simulink model "WinchDynamicsAndControl"  (R2020a)
settings: Solver=FixedStepAuto  StartTime=0.0  StopTime=simInit.TSIM  MaxStep=0.01  RelTol=1e-1
InitFcn:
  | close all
undefined symbols (not defined in the file): constr, DiscIntNeverNeededParam, params, simInit, winchParameter
libraries: simulink x4
Description:
  | % Copyright 2020 Delft University of Technology
  | %
  | % Licensed under the Apache License, Version 2.0 (the "License");
  | % you may not use this file except in compliance with the License.
  | % You may obtain a copy of the License at
  | %
  | %      http://www.apache.org/licenses/LICENSE-2.0
  | %
  | % Unless required by applicable law or agreed to in writing, software
  | % distributed under the License is distributed on an "AS IS" BASIS,
  | % WITHOUT WARRANTIES OR CONDITIONS OF ANY KIND, either express or implied.
  | % See the License for the specific language governing permissions and
  | % limitations under the License.
settings Model: ExtModeTrigDuration=100  Creator=Sebastian  LastModifiedBy=dylaneijkelhof
settings SolverCC: SolverJacobianMethodControl=FullAnalytical
settings DataIOCC: SaveFormat=Array  SaveOutput=off  DSMLogging=off  SaveTime=off  ReturnWorkspaceOutputs=off  StateSaveName=tmp_raccel_xout  SignalLoggingName=logged_signals  LoggingFileName=log
settings OptimizationCC: EfficientMapNaN2IntZero=off  LifeSpan=inf
settings DebuggingCC: ArtificialAlgebraicLoopMsg=none  SaveWithDisabledLinksMsg=none  SaveWithParameterizedLinksMsg=none  MaskedZcDiagnostic=none  IgnoredZcDiagnostic=none  InheritedTsInSrcMsg=none  TasksWithSamePriorityMsg=none  SigSpecEnsureSampleTimeMsg=none  ParameterPrecisionLossMsg=none  UnconnectedInputMsg=none  UnconnectedOutputMsg=none  UnconnectedLineMsg=none  BusObjectLabelMismatch=none  RootOutportRequireBusObject=none  UnknownTsInhSupMsg=none  ModelReferenceDataLoggingMessage=none  ModelReferenceSymbolNameMessage=none  InitInArrayFormatMsg=none  SFUnusedDataAndEventsDiag=none  SFUnexpectedBacktrackingDiag=none  SFInvalidInputDataAccessInChartInitDiag=none  SFNoUnconditionalDefaultTransitionDiag=none  SFTransitionOutsideNaturalParentDiag=none  SFUnreachableExecutionPathDiag=none  SFUndirectedBroadcastEventsDiag=none  SFTransitionActionBeforeConditionDiag=none  SFTemporalDelaySmallerThanSampleTimeDiag=none  SFSelfTransitionDiag=none  SFExecutionAtInitializationDiag=none  SFMachineParentedDataDiag=none  UnitsInconsistencyMsg=none  ArithmeticOperatorsInVariantConditions=warning
settings HardwareCC: TargetBitPerLong=64  TargetBitPerPointer=64  TargetBitPerSizeT=64  TargetBitPerPtrDiffT=64  TargetLongLongMode=on  TargetIntDivRoundTo=Zero  TargetEndianess=LittleEndian  TargetWordSize=64  TargetHWDeviceType=MATLAB Host  ProdEqTarget=off
settings ModelReferenceCC: PropagateSignalLabelsOutOfModel=off
settings SFSimCC: SimUseLocalCustomCode=off  CustomCodeUndefinedFunction=UseInterfaceOnly
settings CodeAppCC: MaxIdLength=128
settings GRTTargetCC: TargetLangStandard=C89/C90 (ANSI)  CombineOutputUpdateFcns=off  GRTInterface=on
settings ConfigComp: CovMetricSettings=dw  CovHtmlReporting=on  CovSaveCumulativeToWorkspaceVar=on  CovSaveSingleToWorkspaceVar=on  CovExternalEMLEnable=off

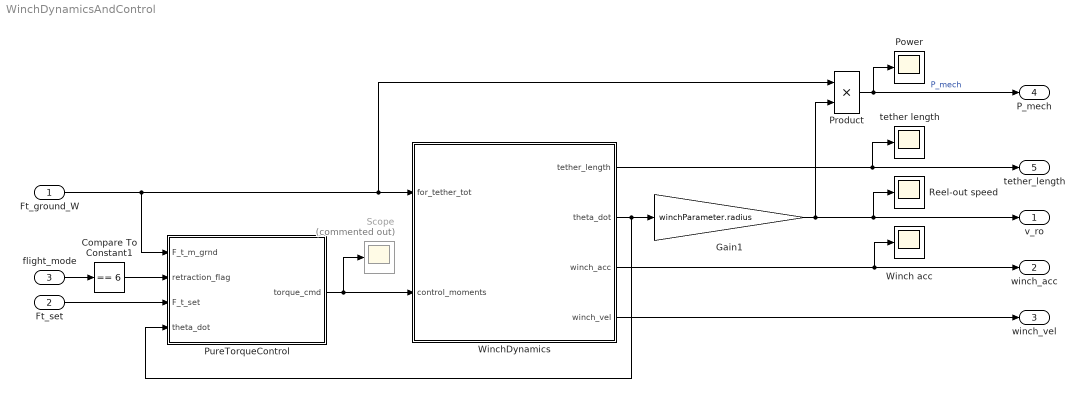
== system WinchDynamicsAndControl ==
  Ft_ground_W : Inport  OutDataTypeStr=double  PortDimensions=1
  Ft_set : Inport  Port=2  OutDataTypeStr=double  PortDimensions=1
  flight_mode : Inport  Port=3  OutDataTypeStr=double  PortDimensions=1
  Compare To Constant1 : simulink/Logic and Bit Operations/Compare To Constant  relop===  const=6  OutDataTypeStr=boolean
  Gain1 : Gain  Gain=winchParameter.radius
  Power : Scope
  Product : Product
  PureTorqueControl : Subsystem
  Reel-out speed : Scope
  Scope : Scope  Commented=on
  Winch acc : Scope
  WinchDynamics : Subsystem
  tether length : Scope
  v_ro : Outport  OutDataTypeStr=double  PortDimensions=1  VectorParamsAs1DForOutWhenUnconnected=off
  winch_acc : Outport  Port=2  OutDataTypeStr=double  PortDimensions=1  VectorParamsAs1DForOutWhenUnconnected=off
  winch_vel : Outport  Port=3  OutDataTypeStr=double  PortDimensions=1  VectorParamsAs1DForOutWhenUnconnected=off
  P_mech : Outport  Port=4  OutDataTypeStr=double  PortDimensions=1  VectorParamsAs1DForOutWhenUnconnected=off
  tether_length : Outport  Port=5  OutDataTypeStr=double  PortDimensions=1  VectorParamsAs1DForOutWhenUnconnected=off
  wires:
  Gain1/1 -> v_ro/1, Reel-out speed/1, Product/2
  WinchDynamics/2(theta_dot) -> Gain1/1, PureTorqueControl/4(theta_dot)
  Ft_ground_W/1 -> Product/1, WinchDynamics/1(for_tether_tot), PureTorqueControl/1(F_t_m_grnd)
  WinchDynamics/4(winch_vel) -> winch_vel/1
  Product/1 -> P_mech/1, Power/1  "P_mech"
  Ft_set/1 -> PureTorqueControl/3(F_t_set)
  flight_mode/1 -> Compare To Constant1/1
  WinchDynamics/3(winch_acc) -> winch_acc/1, Winch acc/1
  WinchDynamics/1(tether_length) -> tether length/1, tether_length/1
  PureTorqueControl/1(torque_cmd) -> Scope/1, WinchDynamics/2(control_moments)
  Compare To Constant1/1 -> PureTorqueControl/2(retraction_flag)

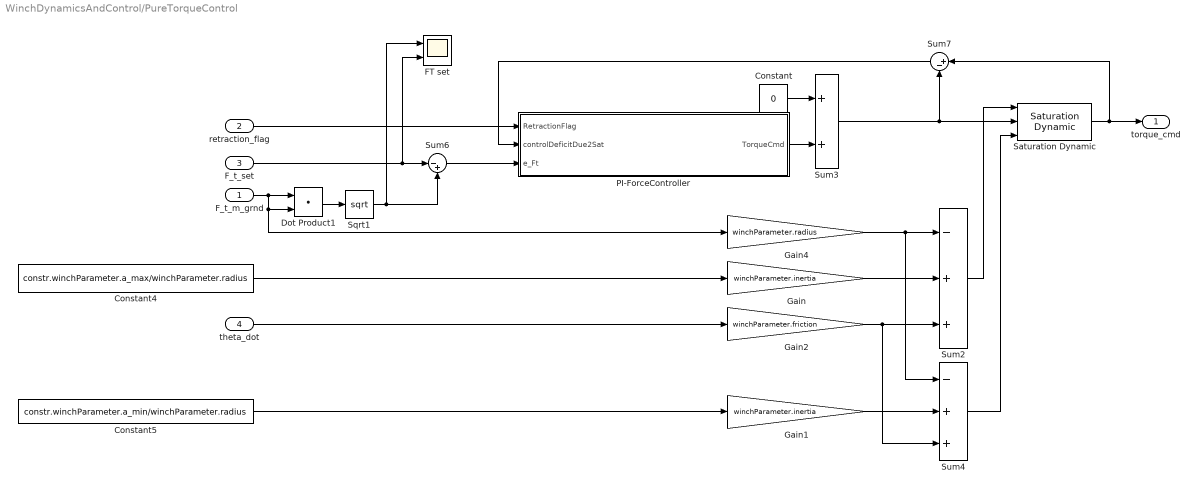
== system WinchDynamicsAndControl/PureTorqueControl ==
  F_t_m_grnd : Inport
  retraction_flag : Inport  Port=2
  F_t_set : Inport  Port=3
  theta_dot : Inport  Port=4
  Constant : Constant  Value=0
  Constant4 : Constant  Value=constr.winchParameter.a_max/winchParameter.radius
  Constant5 : Constant  Value=constr.winchParameter.a_min/winchParameter.radius
  Dot Product1 : DotProduct  InputSameDT=on  OutDataTypeStr=Inherit: Inherit via internal rule
  FT set : Scope  NumInputPorts=2
  Gain : Gain  Gain=winchParameter.inertia
  Gain1 : Gain  Gain=winchParameter.inertia
  Gain2 : Gain  Gain=winchParameter.friction
  Gain4 : Gain  Gain=winchParameter.radius
  PI-ForceController : Subsystem
  Saturation Dynamic : simulink/Discontinuities/Saturation Dynamic  OutMin=[]  OutMax=[]  OutDataTypeStr=Inherit: Same as second input  OutDataType=fixdt(1, 16)  OutScaling=2^-10  DoSatur=off
  Sqrt1 : Sqrt  SaturateOnIntegerOverflow=on
  Sum2 : Sum  Inputs=-++
  Sum3 : Sum
  Sum4 : Sum  Inputs=-++
  Sum6 : Sum  Inputs=|-+
  Sum7 : Sum  Inputs=|+-
  torque_cmd : Outport  VectorParamsAs1DForOutWhenUnconnected=off
  wires:
  Saturation Dynamic/1 -> Sum7/1, torque_cmd/1
  PI-ForceController/1(TorqueCmd) -> Sum3/2
  Sum6/1 -> PI-ForceController/3(e_Ft)
  Sum7/1 -> PI-ForceController/2(controlDeficitDue2Sat)
  retraction_flag/1 -> PI-ForceController/1(RetractionFlag)
  theta_dot/1 -> Gain2/1
  F_t_m_grnd/1 -> Gain4/1, Dot Product1/2, Dot Product1/1
  Dot Product1/1 -> Sqrt1/1
  Sqrt1/1 -> FT set/1, Sum6/2
  Gain2/1 -> Sum2/3, Sum4/3
  Sum3/1 -> Sum7/2, Saturation Dynamic/2
  Sum4/1 -> Saturation Dynamic/3
  Gain1/1 -> Sum4/2
  Constant5/1 -> Gain1/1
  Sum2/1 -> Saturation Dynamic/1
  Gain/1 -> Sum2/2
  Constant4/1 -> Gain/1
  Gain4/1 -> Sum4/1, Sum2/1
  F_t_set/1 -> Sum6/1, FT set/2
  Constant/1 -> Sum3/1

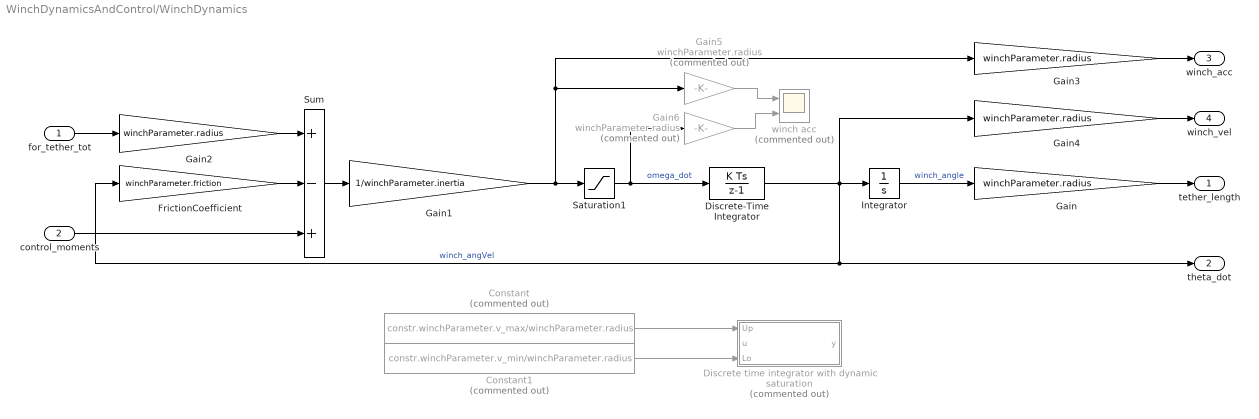
== system WinchDynamicsAndControl/WinchDynamics ==
  for_tether_tot : Inport
  control_moments : Inport  Port=2
  Constant : Constant  Commented=on  Value=constr.winchParameter.v_max/winchParameter.radius
  Constant1 : Constant  Commented=on  Value=constr.winchParameter.v_min/winchParameter.radius
  Discrete time integrator with dynamic saturation : Subsystem  Commented=on  mask{Ts=simInit.dt, K=1}
      mask prompts: Ts "Sample time"; K "Gain"
      mask help: This is an dicrete time integrator with upper and lower bounds.
      mask Display:
      | disp('K Ts\n-----\nz-1')
      | port_label('input', 1, 'Up')
      | port_label('input', 2, 'u')
      | port_label('input', 3, 'Lo')
      | port_label('output', 1, 'y')
  Discrete-Time Integrator : DiscreteIntegrator  SampleTime=simInit.dt  LimitOutput=on  UpperSaturationLimit=constr.winchParameter.v_max/winchParameter.radius  LowerSaturationLimit=constr.winchParameter.v_min/winchParameter.radius  ICPrevOutput=DiscIntNeverNeededParam  ICPrevScaledInput=DiscIntNeverNeededParam
  FrictionCoefficient : Gain  Gain=winchParameter.friction
  Gain{,2..4} (4 alike) : Gain  Gain=winchParameter.radius
  Gain1 : Gain  Gain=1/winchParameter.inertia
  Gain5 : Gain  Commented=on  Gain=winchParameter.radius
  Gain6 : Gain  Commented=on  Gain=winchParameter.radius
  Integrator : Integrator  InitialCondition=simInit.winch_angle_init
  Saturation1 : Saturate  UpperLimit=constr.winchParameter.a_max/winchParameter.radius  LowerLimit=constr.winchParameter.a_min/winchParameter.radius
  Sum : Sum  Inputs=+-+
  winch acc : Scope  Commented=on  NumInputPorts=2
  tether_length : Outport  VectorParamsAs1DForOutWhenUnconnected=off
  theta_dot : Outport  Port=2  VectorParamsAs1DForOutWhenUnconnected=off
  winch_acc : Outport  Port=3  VectorParamsAs1DForOutWhenUnconnected=off
  winch_vel : Outport  Port=4  VectorParamsAs1DForOutWhenUnconnected=off
  wires:
  Constant1/1 -> Discrete time integrator with dynamic saturation/3(Lo)
  Constant/1 -> Discrete time integrator with dynamic saturation/1(Up)
  Gain6/1 -> winch acc/2
  Gain5/1 -> winch acc/1
  Gain3/1 -> winch_acc/1
  Gain4/1 -> winch_vel/1
  Saturation1/1 -> Discrete-Time Integrator/1, Gain6/1  "omega_dot"
  Gain1/1 -> Gain3/1, Gain5/1, Saturation1/1
  for_tether_tot/1 -> Gain2/1
  FrictionCoefficient/1 -> Sum/2
  control_moments/1 -> Sum/3
  Discrete-Time Integrator/1 -> Integrator/1, theta_dot/1, FrictionCoefficient/1, Gain4/1  "winch_angVel"
  Integrator/1 -> Gain/1  "winch_angle"
  Sum/1 -> Gain1/1
  Gain2/1 -> Sum/1
  Gain/1 -> tether_length/1

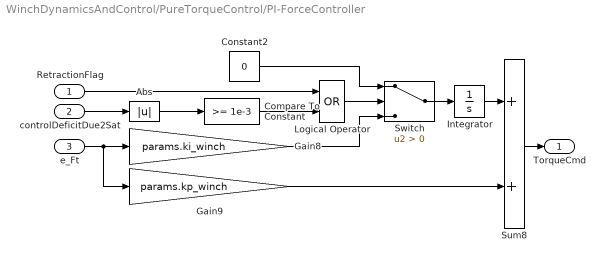
== system WinchDynamicsAndControl/PureTorqueControl/PI-ForceController ==
  RetractionFlag : Inport
  controlDeficitDue2Sat : Inport  Port=2
  e_Ft : Inport  Port=3
  Abs : Abs
  Compare To Constant : simulink/Logic and Bit Operations/Compare To Constant  relop=>=  const=1e-3  OutDataTypeStr=boolean
  Constant2 : Constant  Value=0
  Gain8 : Gain  Gain=params.ki_winch
  Gain9 : Gain  Gain=params.kp_winch
  Integrator : Integrator
  Logical Operator : Logic  Operator=OR  AllPortsSameDT=off  OutDataTypeStr=boolean
  Sum8 : Sum
  Switch : Switch  Criteria=u2 > Threshold
  TorqueCmd : Outport  VectorParamsAs1DForOutWhenUnconnected=off
  wires:
  Logical Operator/1 -> Switch/2
  RetractionFlag/1 -> Logical Operator/1
  controlDeficitDue2Sat/1 -> Abs/1
  e_Ft/1 -> Gain9/1, Gain8/1
  Abs/1 -> Compare To Constant/1
  Integrator/1 -> Sum8/1
  Compare To Constant/1 -> Logical Operator/2
  Gain8/1 -> Switch/3
  Gain9/1 -> Sum8/2
  Constant2/1 -> Switch/1
  Switch/1 -> Integrator/1
  Sum8/1 -> TorqueCmd/1

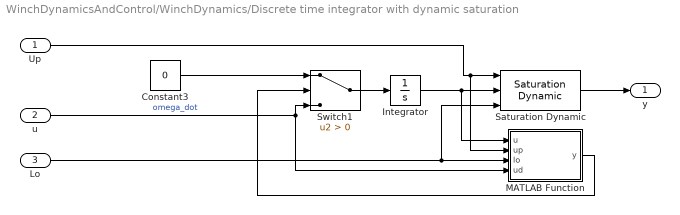
== system WinchDynamicsAndControl/WinchDynamics/Discrete time integrator with dynamic saturation ==
  Up : Inport
  u : Inport  Port=2
  Lo : Inport  Port=3
  Constant3 : Constant  Value=0
  Integrator : Integrator
  MATLAB Function : MATLAB Function  TreatAsAtomicUnit=on
  Saturation Dynamic : simulink/Discontinuities/Saturation Dynamic  OutMin=[]  OutMax=[]  OutDataTypeStr=Inherit: Same as second input  OutDataType=fixdt(1, 16)  OutScaling=2^-10  DoSatur=off
  Switch1 : Switch  Criteria=u2 > Threshold
  y : Outport  VectorParamsAs1DForOutWhenUnconnected=off
  wires:
  Up/1 -> Saturation Dynamic/1, MATLAB Function/2(up)
  Lo/1 -> MATLAB Function/3(lo), Saturation Dynamic/3
  Saturation Dynamic/1 -> y/1
  u/1 -> MATLAB Function/4(ud), Switch1/3  "omega_dot"
  Switch1/1 -> Integrator/1
  MATLAB Function/1(y) -> Switch1/2
  Integrator/1 -> Saturation Dynamic/2, MATLAB Function/1(u)
  Constant3/1 -> Switch1/1

== matlab function WinchDynamicsAndControl/WinchDynamics/Discrete time integrator with dynamic saturation/MATLAB Function ==
  data: u input; y output; up input; lo input; ud input
% Copyright 2020 Delft University of Technology
%
% Licensed under the Apache License, Version 2.0 (the "License");
% you may not use this file except in compliance with the License.
% You may obtain a copy of the License at
%
%      http://www.apache.org/licenses/LICENSE-2.0
%
% Unless required by applicable law or agreed to in writing, software
% distributed under the License is distributed on an "AS IS" BASIS,
% WITHOUT WARRANTIES OR CONDITIONS OF ANY KIND, either express or implied.
% See the License for the specific language governing permissions and
% limitations under the License.

function y = fcn(u, up , lo, ud)
udot = ud;
    if u>up
        y = 1;
        if udot<0
            y=0;
        end
    elseif u<lo
        y = 1;
        if udot>0
            y=0;
        end
    else
        y = 0;
    end
end
